simulink model "CaseMuxThree"  (R2023b)
settings: Solver=VariableStepAuto  StartTime=0.0  StopTime=10.0  RelTol=1e-3
settings Model: Creator=jsonm  LastModifiedBy=jsonm

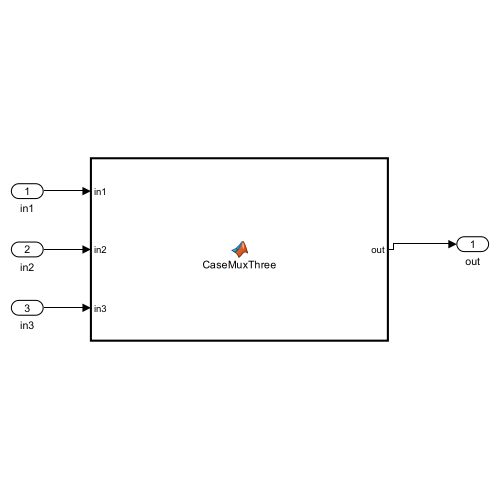
[thumbnail: Simulink's stored preview of the top-level diagram]
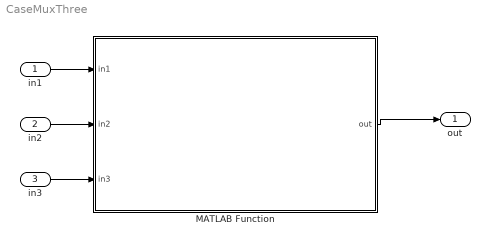
== system CaseMuxThree ==
  in1 : Inport
  in2 : Inport  Port=2
  in3 : Inport  Port=3
  MATLAB Function : MATLAB Function  TreatAsAtomicUnit=on
  out : Outport
  wires:
  in1/1 -> MATLAB Function/1(in1)
  in2/1 -> MATLAB Function/2(in2)
  MATLAB Function/1(out) -> out/1
  in3/1 -> MATLAB Function/3(in3)

== matlab function CaseMuxThree/MATLAB Function ==
  data: in1 input; out output; in2 input; in3 input
function out = CaseMuxThree(in1, in2, in3)

% Method to mux three inputs into one of three possible outputs based on first
% non-negative input
%
% Written by: Darian Muresan
% Modified by: Jason McCauley

if nargin < 1
    in1 = -1;
    in2 = -1;
    in3 = -1;
elseif nargin < 2
    in2 = -1;
    in3 = -1;
elseif nargin < 3
    in3 = -1;
end

if in1 >= 0
    out = in1;
elseif in2 >= 0
    out = in2;
elseif in3 >= 0
    out = in3;
else
    out = -1;
end
